simulink model "SD2231_Lab1_2024_final"  (R2023a)
settings: Solver=FixedStepAuto  StartTime=0.0  StopTime=inf  FixedStep=0.001  RelTol=1e-3  EnableMultiTasking=on
values from neighbouring files (symbols this model uses):
  K_brake = K_brake(3)    [initial_student.m]    (also in initial_student_final.m)
  K_em = K_em(3)    [initial_student.m]    (also in initial_student_final.m)
undefined symbols (not defined in the file or in its folder): DiscIntNeverNeededParam, Veh
libraries: CarMaker4SL x37, simulink x11, SignalEditorBlockLib x2, autolibmappedmotor x2
(part 2 of 4)

== system SD2231_Lab1_2024_final/CarMaker/Your ABS Controller/PID Controller ==
  <FL Braking Slip> : Inport
  <RL Braking Slip> : Inport  Port=2
  <Brake pedal> : Inport  Port=3
  Vehicle_Velocity : Inport  Port=4
  PID_Front_Breaking : Subsystem
  PID_Rear_Breaking : Subsystem
  Sum : Sum  Inputs=|-+
  Sum1 : Sum  Inputs=+-|
  Switch : Switch  Criteria=u2 > Threshold  Threshold=2.5  SaturateOnIntegerOverflow=off  InputSameDT=off
  Switch1 : Switch  Criteria=u2 > Threshold  Threshold=0.05  SaturateOnIntegerOverflow=off  InputSameDT=off
  Switch2 : Switch  Criteria=u2 > Threshold  Threshold=2.5  SaturateOnIntegerOverflow=off  InputSameDT=off
  Switch3 : Switch  Criteria=u2 > Threshold  Threshold=0.05  SaturateOnIntegerOverflow=off  InputSameDT=off
  Front_Braking : Outport
  Rear_Braking : Outport  Port=2
  wires:
  <FL Braking Slip>/1 -> PID_Front_Breaking/1(In1), Switch1/2
  PID_Front_Breaking/1(Out1) -> Sum/1
  <Brake pedal>/1 -> Switch3/3, Switch2/3, Switch1/3, Switch/3, Sum/2, Sum1/1
  <RL Braking Slip>/1 -> PID_Rear_Breaking/1(In1), Switch3/2
  Sum/1 -> Switch1/1
  Switch1/1 -> Switch/1
  Switch/1 -> Front_Braking/1
  Vehicle_Velocity/1 -> Switch/2, Switch2/2
  Switch3/1 -> Switch2/1
  Switch2/1 -> Rear_Braking/1
  Sum1/1 -> Switch3/1
  PID_Rear_Breaking/1(Out1) -> Sum1/2

== system SD2231_Lab1_2024_final/CarMaker/Your ABS Controller/PID Controller Advanced filter ==
  <FL Braking Slip> : Inport
  <RL Braking Slip> : Inport  Port=2
  <Brake pedal> : Inport  Port=3
  Vehicle_Velocity : Inport  Port=4
  PID_Front_Breaking : Subsystem
  PID_Rear_Breaking : Subsystem
  Sum : Sum  Inputs=|-+
  Sum1 : Sum  Inputs=+-|
  Switch : Switch  Criteria=u2 > Threshold  Threshold=2.5  SaturateOnIntegerOverflow=off  InputSameDT=off
  Switch1 : Switch  Criteria=u2 > Threshold  Threshold=0.05  SaturateOnIntegerOverflow=off  InputSameDT=off
  Switch2 : Switch  Criteria=u2 > Threshold  Threshold=2.5  SaturateOnIntegerOverflow=off  InputSameDT=off
  Switch3 : Switch  Criteria=u2 > Threshold  Threshold=0.05  SaturateOnIntegerOverflow=off  InputSameDT=off
  Front_Braking : Outport
  Rear_Braking : Outport  Port=2
  wires:
  <FL Braking Slip>/1 -> PID_Front_Breaking/1(In1), Switch1/2
  PID_Front_Breaking/1(Out1) -> Sum/1
  <Brake pedal>/1 -> Switch3/3, Switch2/3, Switch1/3, Switch/3, Sum/2, Sum1/1
  <RL Braking Slip>/1 -> PID_Rear_Breaking/1(In1), Switch3/2
  Sum/1 -> Switch1/1
  Switch1/1 -> Switch/1
  Switch/1 -> Front_Braking/1
  Vehicle_Velocity/1 -> Switch/2, Switch2/2
  Switch3/1 -> Switch2/1
  Switch2/1 -> Rear_Braking/1
  Sum1/1 -> Switch3/1
  PID_Rear_Breaking/1(Out1) -> Sum1/2

== system SD2231_Lab1_2024_final/CarMaker/Your ABS Controller/PID Controller windup ==
  <FL Braking Slip> : Inport
  <RL Braking Slip> : Inport  Port=2
  <Brake pedal> : Inport  Port=3
  Vehicle_Velocity : Inport  Port=4
  Minus : Sum  Inputs=+-
  Minus1 : Sum  Inputs=+-
  PID_Front_Breaking : Subsystem
  PID_Rear_Breaking : Subsystem
  Saturation : Saturate  UpperLimit=1  LowerLimit=0
  Saturation1 : Saturate  UpperLimit=1  LowerLimit=0
  Sum : Sum  Inputs=|-+
  Sum1 : Sum  Inputs=+-|
  Switch : Switch  Criteria=u2 > Threshold  Threshold=2.5  SaturateOnIntegerOverflow=off  InputSameDT=off
  Switch1 : Switch  Criteria=u2 > Threshold  Threshold=0.05  SaturateOnIntegerOverflow=off  InputSameDT=off
  Switch2 : Switch  Criteria=u2 > Threshold  Threshold=2.5  SaturateOnIntegerOverflow=off  InputSameDT=off
  Switch3 : Switch  Criteria=u2 > Threshold  Threshold=0.05  SaturateOnIntegerOverflow=off  InputSameDT=off
  Front_Braking : Outport
  Rear_Braking : Outport  Port=2
  wires:
  <FL Braking Slip>/1 -> PID_Front_Breaking/1(In1), Switch1/2
  PID_Front_Breaking/1(Out1) -> Sum/1
  <Brake pedal>/1 -> Switch3/3, Switch2/3, Switch1/3, Switch/3, Sum/2, Sum1/1
  <RL Braking Slip>/1 -> PID_Rear_Breaking/1(In1), Switch3/2
  Switch1/1 -> Switch/1
  Switch/1 -> Front_Braking/1
  Vehicle_Velocity/1 -> Switch/2, Switch2/2
  Switch3/1 -> Switch2/1
  Switch2/1 -> Rear_Braking/1
  Sum1/1 -> Saturation1/1, Minus1/2, Switch3/1
  PID_Rear_Breaking/1(Out1) -> Sum1/2
  Saturation/1 -> Minus/1
  Sum/1 -> Saturation/1, Minus/2, Switch1/1
  Minus/1 -> PID_Front_Breaking/2(In2)
  Saturation1/1 -> Minus1/1
  Minus1/1 -> PID_Rear_Breaking/2(In2)

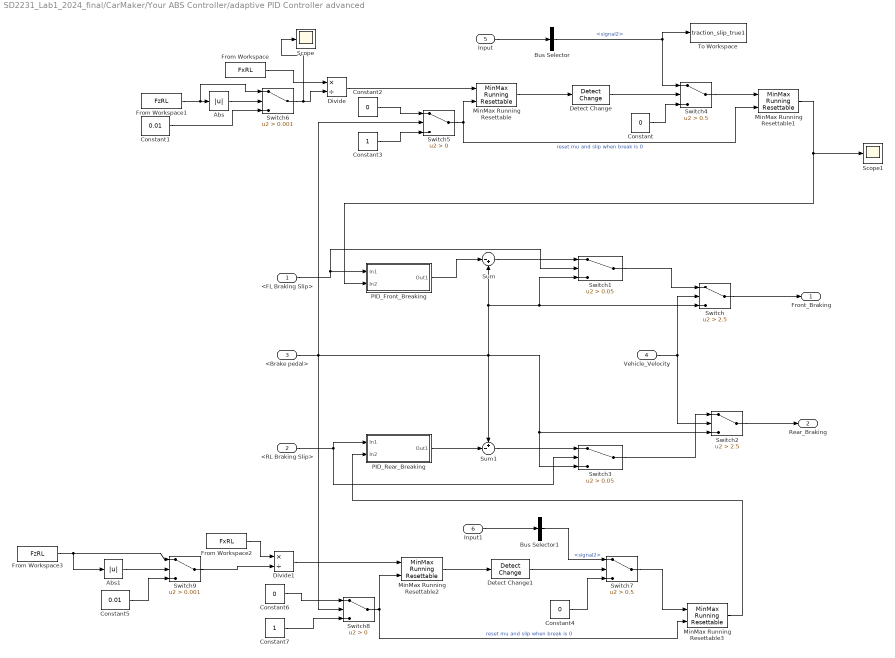
== system SD2231_Lab1_2024_final/CarMaker/Your ABS Controller/adaptive PID Controller advanced ==
  <FL Braking Slip> : Inport
  <RL Braking Slip> : Inport  Port=2
  <Brake pedal> : Inport  Port=3
  Vehicle_Velocity : Inport  Port=4
  Input : Inport  Port=5
  Input1 : Inport  Port=6
  Abs : Abs  SaturateOnIntegerOverflow=off
  Abs1 : Abs  SaturateOnIntegerOverflow=off
  Bus Selector : BusSelector  OutputSignals=signal2
  Bus Selector1 : BusSelector  OutputSignals=signal2
  Constant{,2,4,6} (4 alike) : Constant  Value=0
  Constant1 : Constant  Value=0.01
  Constant3 : Constant
  Constant5 : Constant  Value=0.01
  Constant7 : Constant
  Detect Change : simulink/Logic and Bit Operations/Detect Change  vinit=0  OutDataTypeStr=boolean
  Detect Change1 : simulink/Logic and Bit Operations/Detect Change  vinit=0  OutDataTypeStr=boolean
  Divide : Product  Inputs=*/
  Divide1 : Product  Inputs=*/
  From Workspace : FromWorkspace  VariableName=FxRL
  From Workspace1 : FromWorkspace  VariableName=FzRL
  From Workspace2 : FromWorkspace  VariableName=FxRL
  From Workspace3 : FromWorkspace  VariableName=FzRL
  MinMax Running Resettable : simulink/Math Operations/MinMax Running Resettable  Function=max  vinit=0.0
  MinMax Running Resettable1 : simulink/Math Operations/MinMax Running Resettable  Function=max  vinit=0.1
  MinMax Running Resettable2 : simulink/Math Operations/MinMax Running Resettable  Function=max  vinit=0.0
  MinMax Running Resettable3 : simulink/Math Operations/MinMax Running Resettable  Function=max  vinit=0.1
  PID_Front_Breaking : Subsystem
  PID_Rear_Breaking : Subsystem
  Scope : Scope
  Scope1 : Scope
  Sum : Sum  Inputs=|-+
  Sum1 : Sum  Inputs=+-|
  Switch : Switch  Criteria=u2 > Threshold  Threshold=2.5  SaturateOnIntegerOverflow=off  InputSameDT=off
  Switch1 : Switch  Criteria=u2 > Threshold  Threshold=0.05  SaturateOnIntegerOverflow=off  InputSameDT=off
  Switch2 : Switch  Criteria=u2 > Threshold  Threshold=2.5  SaturateOnIntegerOverflow=off  InputSameDT=off
  Switch3 : Switch  Criteria=u2 > Threshold  Threshold=0.05  SaturateOnIntegerOverflow=off  InputSameDT=off
  Switch4 : Switch  Criteria=u2 > Threshold  Threshold=0.5  SaturateOnIntegerOverflow=off  InputSameDT=off
  Switch5 : Switch  Criteria=u2 > Threshold  SaturateOnIntegerOverflow=off  InputSameDT=off
  Switch6 : Switch  Criteria=u2 > Threshold  Threshold=0.001  SaturateOnIntegerOverflow=off  InputSameDT=off
  Switch7 : Switch  Criteria=u2 > Threshold  Threshold=0.5  SaturateOnIntegerOverflow=off  InputSameDT=off
  Switch8 : Switch  Criteria=u2 > Threshold  SaturateOnIntegerOverflow=off  InputSameDT=off
  Switch9 : Switch  Criteria=u2 > Threshold  Threshold=0.001  SaturateOnIntegerOverflow=off  InputSameDT=off
  To Workspace : ToWorkspace  VariableName=traction_slip_true1  SaveFormat=Timeseries  SampleTime=-1
  Front_Braking : Outport
  Rear_Braking : Outport  Port=2
  wires:
  <FL Braking Slip>/1 -> PID_Front_Breaking/1(In1), Switch1/2
  PID_Front_Breaking/1(Out1) -> Sum/1
  <RL Braking Slip>/1 -> PID_Rear_Breaking/1(In1), Switch3/2
  Sum/1 -> Switch1/1
  Switch1/1 -> Switch/1
  Switch/1 -> Front_Braking/1
  Vehicle_Velocity/1 -> Switch/2, Switch2/2
  Switch3/1 -> Switch2/1
  Switch2/1 -> Rear_Braking/1
  Sum1/1 -> Switch3/1
  PID_Rear_Breaking/1(Out1) -> Sum1/2
  Abs/1 -> Switch6/2
  Switch6/1 -> Scope/1, Divide/2
  From Workspace1/1 -> Switch6/1, Abs/1
  Input/1 -> Bus Selector/1
  Constant/1 -> Switch4/3
  Bus Selector/1 -> To Workspace/1, Switch4/1  "<signal2>"
  From Workspace/1 -> Divide/1
  MinMax Running Resettable1/1 -> PID_Front_Breaking/2(In2), Scope1/1
  Constant1/1 -> Switch6/3
  MinMax Running Resettable/1 -> Detect Change/1
  Switch4/1 -> MinMax Running Resettable1/1
  Constant3/1 -> Switch5/3
  Switch5/1 -> MinMax Running Resettable/2, MinMax Running Resettable1/2  "reset mu and slip when break is 0"
  Constant2/1 -> Switch5/1
  Divide/1 -> MinMax Running Resettable/1
  Detect Change/1 -> Switch4/2
  Switch9/1 -> Divide1/2
  Abs1/1 -> Switch9/2
  Divide1/1 -> MinMax Running Resettable2/1
  Detect Change1/1 -> Switch7/2
  MinMax Running Resettable2/1 -> Detect Change1/1
  Constant7/1 -> Switch8/3
  Constant5/1 -> Switch9/3
  Switch7/1 -> MinMax Running Resettable3/1
  Constant6/1 -> Switch8/1
  Switch8/1 -> MinMax Running Resettable2/2, MinMax Running Resettable3/2  "reset mu and slip when break is 0"
  From Workspace2/1 -> Divide1/1
  Bus Selector1/1 -> Switch7/1  "<signal2>"
  Constant4/1 -> Switch7/3
  Input1/1 -> Bus Selector1/1
  <Brake pedal>/1 -> Switch5/2, Switch3/3, Switch2/3, Switch1/3, Switch/3, Sum/2, Sum1/1, Switch8/2
  From Workspace3/1 -> Abs1/1, Switch9/1
  MinMax Running Resettable3/1 -> PID_Rear_Breaking/2(In2)

== system SD2231_Lab1_2024_final/CarMaker/Your Traction Controller/P Controller ==
  <RL traction slip> : Inport
  <Throttle> : Inport  Port=2
  Vehicle_Velocity : Inport  Port=3
  P_Front_Breaking : Subsystem
  Sum : Sum  Inputs=|-+
  Switch : Switch  Criteria=u2 > Threshold  Threshold=2.5  SaturateOnIntegerOverflow=off  InputSameDT=off
  Switch1 : Switch  Criteria=u2 > Threshold  Threshold=0.3  SaturateOnIntegerOverflow=off  InputSameDT=off
  Throttle : Outport
  wires:
  <RL traction slip>/1 -> P_Front_Breaking/1(In1), Switch1/2
  P_Front_Breaking/1(Out1) -> Sum/1
  <Throttle>/1 -> Switch1/3, Switch/3, Sum/2
  Sum/1 -> Switch1/1
  Switch1/1 -> Switch/1
  Switch/1 -> Throttle/1
  Vehicle_Velocity/1 -> Switch/2

== system SD2231_Lab1_2024_final/CarMaker/Your Traction Controller/PD Controller ==
  <RL traction slip> : Inport
  <Throttle> : Inport  Port=2
  Vehicle_Velocity : Inport  Port=3
  P_Front_Breaking : Subsystem
  Sum : Sum  Inputs=|-+
  Switch : Switch  Criteria=u2 > Threshold  Threshold=2.5  SaturateOnIntegerOverflow=off  InputSameDT=off
  Switch1 : Switch  Criteria=u2 > Threshold  Threshold=0.3  SaturateOnIntegerOverflow=off  InputSameDT=off
  Throttle : Outport
  wires:
  <RL traction slip>/1 -> P_Front_Breaking/1(In1), Switch1/2
  P_Front_Breaking/1(Out1) -> Sum/1
  <Throttle>/1 -> Switch1/3, Switch/3, Sum/2
  Sum/1 -> Switch1/1
  Switch1/1 -> Switch/1
  Switch/1 -> Throttle/1
  Vehicle_Velocity/1 -> Switch/2

== system SD2231_Lab1_2024_final/CarMaker/Your Traction Controller/PI Controller ==
  <RL traction slip> : Inport
  <Throttle> : Inport  Port=2
  Vehicle_Velocity : Inport  Port=3
  P_Front_Breaking : Subsystem
  Sum : Sum  Inputs=|-+
  Switch : Switch  Criteria=u2 > Threshold  Threshold=2.5  SaturateOnIntegerOverflow=off  InputSameDT=off
  Switch1 : Switch  Criteria=u2 > Threshold  Threshold=0.2  SaturateOnIntegerOverflow=off  InputSameDT=off
  Throttle : Outport
  wires:
  <RL traction slip>/1 -> P_Front_Breaking/1(In1), Switch1/2
  P_Front_Breaking/1(Out1) -> Sum/1
  <Throttle>/1 -> Switch1/3, Switch/3, Sum/2
  Sum/1 -> Switch1/1
  Switch1/1 -> Switch/1
  Switch/1 -> Throttle/1
  Vehicle_Velocity/1 -> Switch/2

== system SD2231_Lab1_2024_final/CarMaker/Your Traction Controller/PID Controller ==
  <RL traction slip> : Inport
  <Throttle> : Inport  Port=2
  Vehicle_Velocity : Inport  Port=3
  P_Front_Breaking : Subsystem
  Sum : Sum  Inputs=|-+
  Switch : Switch  Criteria=u2 > Threshold  Threshold=2.5  SaturateOnIntegerOverflow=off  InputSameDT=off
  Switch1 : Switch  Criteria=u2 > Threshold  Threshold=0.2  SaturateOnIntegerOverflow=off  InputSameDT=off
  Throttle : Outport
  wires:
  <RL traction slip>/1 -> P_Front_Breaking/1(In1), Switch1/2
  P_Front_Breaking/1(Out1) -> Sum/1
  <Throttle>/1 -> Switch1/3, Switch/3, Sum/2
  Sum/1 -> Switch1/1
  Switch1/1 -> Switch/1
  Switch/1 -> Throttle/1
  Vehicle_Velocity/1 -> Switch/2

== system SD2231_Lab1_2024_final/CarMaker/Your Traction Controller/PID Controller Advanced anti-windup ==
  <RL traction slip> : Inport
  <Throttle> : Inport  Port=2
  Vehicle_Velocity : Inport  Port=3
  Minus : Sum  Inputs=+-
  P_Front_Breaking : Subsystem
  Saturation : Saturate  UpperLimit=1  LowerLimit=0
  Sum : Sum  Inputs=|-+
  Switch : Switch  Criteria=u2 > Threshold  Threshold=2.5  SaturateOnIntegerOverflow=off  InputSameDT=off
  Switch1 : Switch  Criteria=u2 > Threshold  Threshold=0.2  SaturateOnIntegerOverflow=off  InputSameDT=off
  Throttle : Outport
  wires:
  <RL traction slip>/1 -> P_Front_Breaking/1(In1), Switch1/2
  P_Front_Breaking/1(Out1) -> Sum/1
  <Throttle>/1 -> Switch1/3, Switch/3, Sum/2
  Sum/1 -> Minus/2, Switch1/1, Saturation/1
  Switch1/1 -> Switch/1
  Switch/1 -> Throttle/1
  Vehicle_Velocity/1 -> Switch/2
  Saturation/1 -> Minus/1
  Minus/1 -> P_Front_Breaking/2(In2)

== system SD2231_Lab1_2024_final/CarMaker/Your Traction Controller/PID Controller Advanced_filter ==
  <RL traction slip> : Inport
  <Throttle> : Inport  Port=2
  Vehicle_Velocity : Inport  Port=3
  P_Front_Breaking : Subsystem
  Sum : Sum  Inputs=|-+
  Switch : Switch  Criteria=u2 > Threshold  Threshold=2.5  SaturateOnIntegerOverflow=off  InputSameDT=off
  Switch1 : Switch  Criteria=u2 > Threshold  Threshold=0.2  SaturateOnIntegerOverflow=off  InputSameDT=off
  Throttle : Outport
  wires:
  <RL traction slip>/1 -> P_Front_Breaking/1(In1), Switch1/2
  P_Front_Breaking/1(Out1) -> Sum/1
  <Throttle>/1 -> Switch1/3, Switch/3, Sum/2
  Sum/1 -> Switch1/1
  Switch1/1 -> Switch/1
  Switch/1 -> Throttle/1
  Vehicle_Velocity/1 -> Switch/2

== system SD2231_Lab1_2024_final/CarMaker/Your Traction Controller/adaptive PID Controller Advanced ==
  <RL traction slip> : Inport
  <Throttle> : Inport  Port=2
  Vehicle_Velocity : Inport  Port=3
  Input : Inport  Port=4
  Abs : Abs  SaturateOnIntegerOverflow=off
  Bus Selector : BusSelector  OutputSignals=signal1
  Constant : Constant  Value=0
  Constant1 : Constant  Value=0.01
  Constant2 : Constant  Value=0
  Constant3 : Constant
  Detect Change : simulink/Logic and Bit Operations/Detect Change  vinit=0  OutDataTypeStr=boolean
  Divide : Product  Inputs=*/
  From Workspace : FromWorkspace  VariableName=FxRL
  From Workspace1 : FromWorkspace  VariableName=FzRL
  MinMax Running Resettable : simulink/Math Operations/MinMax Running Resettable  Function=max  vinit=0.0
  MinMax Running Resettable1 : simulink/Math Operations/MinMax Running Resettable  Function=max  vinit=0.1
  PID_Rear_Thrust : Subsystem
  Scope : Scope
  Scope1 : Scope
  Scope2 : Scope
  Sum : Sum  Inputs=|-+
  Switch : Switch  Criteria=u2 > Threshold  Threshold=2.5  SaturateOnIntegerOverflow=off  InputSameDT=off
  Switch1 : Switch  Criteria=u2 > Threshold  Threshold=0.2  SaturateOnIntegerOverflow=off  InputSameDT=off
  Switch2 : Switch  Criteria=u2 > Threshold  Threshold=0.5  SaturateOnIntegerOverflow=off  InputSameDT=off
  Switch3 : Switch  Criteria=u2 > Threshold  SaturateOnIntegerOverflow=off  InputSameDT=off
  Switch4 : Switch  Criteria=u2 > Threshold  Threshold=0.001  SaturateOnIntegerOverflow=off  InputSameDT=off
  To Workspace : ToWorkspace  VariableName=traction_slip_true  SaveFormat=Timeseries  SampleTime=-1
  To Workspace1 : ToWorkspace  VariableName=traction_slip_best  SaveFormat=Timeseries  SampleTime=-1
  Throttle : Outport
  wires:
  <RL traction slip>/1 -> Switch1/2, PID_Rear_Thrust/1(In1)
  PID_Rear_Thrust/1(Out1) -> Sum/1
  <Throttle>/1 -> Switch1/3, Switch/3, Sum/2, Switch3/2
  Sum/1 -> Switch1/1
  Switch1/1 -> Switch/1
  Switch/1 -> Throttle/1
  Vehicle_Velocity/1 -> Switch/2
  From Workspace/1 -> Divide/1
  Divide/1 -> MinMax Running Resettable/1
  MinMax Running Resettable/1 -> Detect Change/1
  Detect Change/1 -> Switch2/2
  Switch2/1 -> MinMax Running Resettable1/1
  Input/1 -> Bus Selector/1
  Bus Selector/1 -> To Workspace/1, Scope1/1, Switch2/1  "<signal1>"
  MinMax Running Resettable1/1 -> To Workspace1/1, PID_Rear_Thrust/2(adaptive reference), Scope2/1
  Constant2/1 -> Switch3/1
  Constant3/1 -> Switch3/3
  Switch3/1 -> MinMax Running Resettable/2, MinMax Running Resettable1/2  "reset mu and slip when throttle is 0"
  Constant/1 -> Switch2/3
  Switch4/1 -> Scope/1, Divide/2
  From Workspace1/1 -> Switch4/1, Abs/1
  Abs/1 -> Switch4/2
  Constant1/1 -> Switch4/3

== system SD2231_Lab1_2024_final/CarMaker/IPG Vehicle/Brake/CreateBus Vhcl.Wheel.PT ==
  In : Inport
  BusCreator1 : BusCreator  Inputs=20
  Demux1 : Demux  Outputs=20
      settings: DisplayOption=none
  Out : Outport  VectorParamsAs1DForOutWhenUnconnected=off
  wires:
  Demux1/20 -> BusCreator1/20  "Vhcl Trq_DriveSrc_trg d3"
  Demux1/19 -> BusCreator1/19  "Vhcl Trq_DriveSrc_trg d2"
  Demux1/18 -> BusCreator1/18  "Vhcl Trq_DriveSrc_trg d1"
  Demux1/17 -> BusCreator1/17  "Vhcl Trq_DriveSrc_trg d0"
  Demux1/16 -> BusCreator1/16  "Vhcl Wheel RR WhlBearing"
  Demux1/15 -> BusCreator1/15  "Vhcl Wheel RR Trq_T2W"
  Demux1/14 -> BusCreator1/14  "Vhcl Wheel RR Trq_BrakeReg_trg"
  Demux1/13 -> BusCreator1/13  "Vhcl Wheel RR Trq_Brake"
  Demux1/12 -> BusCreator1/12  "Vhcl Wheel RL WhlBearing"
  Demux1/11 -> BusCreator1/11  "Vhcl Wheel RL Trq_T2W"
  Demux1/10 -> BusCreator1/10  "Vhcl Wheel RL Trq_BrakeReg_trg"
  Demux1/9 -> BusCreator1/9  "Vhcl Wheel RL Trq_Brake"
  Demux1/8 -> BusCreator1/8  "Vhcl Wheel FR WhlBearing"
  Demux1/7 -> BusCreator1/7  "Vhcl Wheel FR Trq_T2W"
  Demux1/6 -> BusCreator1/6  "Vhcl Wheel FR Trq_BrakeReg_trg"
  Demux1/5 -> BusCreator1/5  "Vhcl Wheel FR Trq_Brake"
  Demux1/4 -> BusCreator1/4  "Vhcl Wheel FL WhlBearing"
  Demux1/3 -> BusCreator1/3  "Vhcl Wheel FL Trq_T2W"
  Demux1/2 -> BusCreator1/2  "Vhcl Wheel FL Trq_BrakeReg_trg"
  Demux1/1 -> BusCreator1/1  "Vhcl Wheel FL Trq_Brake"
  BusCreator1/1 -> Out/1
  In/1 -> Demux1/1

== system SD2231_Lab1_2024_final/CarMaker/IPG Vehicle/Brake/UserDefinedBrakingSystem ==
  note: Please note: Influence of DrivMan.Handbrake on the braking
      | torques (Brake IF Trq_XX signals) is ignored in this example.
  SD2231.Data : Inport
  Bus Creator2 : BusCreator  Inputs=16
  Bus Selector : BusSelector  OutputSignals=FLBrakeAdjust,FRBrakeAdjust,RLBrakeAdjust,RRBrakeAdjust
  Constant : Constant  Value=0
  NOTSET : Constant  Value=-99999
  Subsystem : Subsystem
  Subsystem1 : Subsystem
  Subsystem2 : Subsystem
  Subsystem3 : Subsystem
  Brake.IF.Out : Outport  VectorParamsAs1DForOutWhenUnconnected=off
  wires:
  SD2231.Data/1 -> Bus Selector/1
  Bus Creator2/1 -> Brake.IF.Out/1
  Constant/1 -> Bus Creator2/10, Bus Creator2/5, Bus Creator2/6, Bus Creator2/7, Bus Creator2/8, Bus Creator2/9, Bus Creator2/11, Bus Creator2/12
  NOTSET/1 -> Bus Creator2/13, Bus Creator2/14, Bus Creator2/15, Bus Creator2/16
  Subsystem/1(FL brake force) -> Bus Creator2/1
  Bus Selector/1 -> Subsystem/1(FLBrakeAdjust)  "<FLBrakeAdjust>"
  Subsystem1/1(FR brake force) -> Bus Creator2/2
  Subsystem2/1(RL brake force) -> Bus Creator2/3
  Subsystem3/1(RR brake force) -> Bus Creator2/4
  Bus Selector/2 -> Subsystem1/1(FRBrakeAdjust)  "<FRBrakeAdjust>"
  Bus Selector/3 -> Subsystem2/1(RLBrakeAdjust)  "<RLBrakeAdjust>"
  Bus Selector/4 -> Subsystem3/1(RRBrakeAdjust)  "<RRBrakeAdjust>"

== system SD2231_Lab1_2024_final/CarMaker/IPG Vehicle/CarAndTrailer/CarAndTrailerUpd ==
  Sync_In : Inport
  Vhcl.Steering : Inport  Port=2
  Vhcl.Motion : Inport  Port=3
  Vhcl.PoI : Inport  Port=4
  Vhcl.Wheel.FL : Inport  Port=5
  Vhcl.Wheel.FR : Inport  Port=6
  Vhcl.Wheel.RL : Inport  Port=7
  Vhcl.Wheel.RR : Inport  Port=8
  Car.Hitch.FrcTrq : Inport  Port=9
  Vhcl.Fr1A : Inport  Port=10
  CarAndTrailerUpd : S-Function  FunctionName=CM_Sfun  Parameters='CarAndTrUpd'  SFunctionDeploymentMode=off  EnableBusSupport=off
  CreateBus Brake.IF.In : Subsystem
  Sync_Out : Outport  VectorParamsAs1DForOutWhenUnconnected=off
  Brake.IF.In : Outport  Port=2  VectorParamsAs1DForOutWhenUnconnected=off
  wires:
  Vhcl.Fr1A/1 -> CarAndTrailerUpd/10  "user vehicle only"
  Vhcl.Steering/1 -> CarAndTrailerUpd/2
  Vhcl.Motion/1 -> CarAndTrailerUpd/3
  Vhcl.PoI/1 -> CarAndTrailerUpd/4
  Vhcl.Wheel.FL/1 -> CarAndTrailerUpd/5
  Vhcl.Wheel.FR/1 -> CarAndTrailerUpd/6
  Car.Hitch.FrcTrq/1 -> CarAndTrailerUpd/9
  Vhcl.Wheel.RR/1 -> CarAndTrailerUpd/8
  Vhcl.Wheel.RL/1 -> CarAndTrailerUpd/7
  CarAndTrailerUpd/2 -> CreateBus Brake.IF.In/1(In)
  CreateBus Brake.IF.In/1(Out) -> Brake.IF.In/1
  CarAndTrailerUpd/1 -> Sync_Out/1
  Sync_In/1 -> CarAndTrailerUpd/1

== system SD2231_Lab1_2024_final/CarMaker/IPG Vehicle/CarAndTrailer/Forces ==
  Sync_In : Inport
  TireFL_In : Inport  Port=2
  TireFR_In : Inport  Port=3
  TireRL_In : Inport  Port=4
  TireRR_In : Inport  Port=5
  lSpring : Inport  Port=6
  vDamp : Inport  Port=7
  lStabi : Inport  Port=8
  lBuf : Inport  Port=9
  External Suspension Forces : Subsystem
  Suspension Forces : Subsystem
  Tires : Subsystem
  Vehicle Forces : Subsystem
  Sync_Out : Outport  VectorParamsAs1DForOutWhenUnconnected=off
  Car.Virtual : Outport  Port=2  VectorParamsAs1DForOutWhenUnconnected=off
  Car.Aero : Outport  Port=3  VectorParamsAs1DForOutWhenUnconnected=off
  Car.Load : Outport  Port=4  VectorParamsAs1DForOutWhenUnconnected=off
  TireFL_Out : Outport  Port=5  VectorParamsAs1DForOutWhenUnconnected=off
  TireFR_Out : Outport  Port=6  VectorParamsAs1DForOutWhenUnconnected=off
  TireRL_Out : Outport  Port=7  VectorParamsAs1DForOutWhenUnconnected=off
  TireRR_Out : Outport  Port=8  VectorParamsAs1DForOutWhenUnconnected=off
  FSpring_ext : Outport  Port=9  VectorParamsAs1DForOutWhenUnconnected=off
  FDamp_ext : Outport  Port=10  VectorParamsAs1DForOutWhenUnconnected=off
  FStabi_ext : Outport  Port=11  VectorParamsAs1DForOutWhenUnconnected=off
  FBuf_ext : Outport  Port=12  VectorParamsAs1DForOutWhenUnconnected=off
  wires:
  lBuf/1 -> External Suspension Forces/5(lBuf), Suspension Forces/5(lBuf)
  lStabi/1 -> External Suspension Forces/4(lStabi), Suspension Forces/4(lStabi)
  vDamp/1 -> External Suspension Forces/3(vDamp), Suspension Forces/3(vDamp)
  Tires/4(TireRR_Out) -> TireRR_Out/1
  Tires/3(TireRL_Out) -> TireRL_Out/1
  Tires/2(TireFR_Out) -> TireFR_Out/1
  Tires/1(TireFL_Out) -> TireFL_Out/1
  TireRR_In/1 -> Tires/5(TireRR_In)
  TireRL_In/1 -> Tires/4(TireRL_In)
  TireFR_In/1 -> Tires/3(TireFR_In)
  TireFL_In/1 -> Tires/2(TireFL_In)
  External Suspension Forces/4(FBuf_ext) -> FBuf_ext/1
  Sync_In/1 -> External Suspension Forces/1(Sync_In), Tires/1(Sync_In), Vehicle Forces/1(Sync_In)
  Vehicle Forces/1(Sync_Out) -> Suspension Forces/1(Sync_In)
  Vehicle Forces/2(Car.Virtual) -> Car.Virtual/1
  Vehicle Forces/3(Car.Aero) -> Car.Aero/1
  Vehicle Forces/4(Car.Load) -> Car.Load/1
  lSpring/1 -> External Suspension Forces/2(lSpring), Suspension Forces/2(lSpring)
  External Suspension Forces/2(FDamp_ext) -> FDamp_ext/1
  External Suspension Forces/3(FStabi_ext) -> FStabi_ext/1
  External Suspension Forces/1(FSpring_ext) -> FSpring_ext/1
  Suspension Forces/1(Sync_Out) -> Sync_Out/1

== system SD2231_Lab1_2024_final/CarMaker/IPG Vehicle/CarAndTrailer/Kinematics ==
  Sync_In : Inport
  Steer.IF : Inport  Port=2
  Kinematics : S-Function  FunctionName=CM_Sfun  Parameters='Kinematics'  SFunctionDeploymentMode=off  EnableBusSupport=off
  Sync_Out : Outport  VectorParamsAs1DForOutWhenUnconnected=off
  TireFL_In : Outport  Port=2  VectorParamsAs1DForOutWhenUnconnected=off
  TireFR_In : Outport  Port=3  VectorParamsAs1DForOutWhenUnconnected=off
  TireRL_In : Outport  Port=4  VectorParamsAs1DForOutWhenUnconnected=off
  TireRR_In : Outport  Port=5  VectorParamsAs1DForOutWhenUnconnected=off
  lSpring : Outport  Port=6  VectorParamsAs1DForOutWhenUnconnected=off
  vDamp : Outport  Port=7  VectorParamsAs1DForOutWhenUnconnected=off
  lStabi : Outport  Port=8  VectorParamsAs1DForOutWhenUnconnected=off
  lBuf : Outport  Port=9  VectorParamsAs1DForOutWhenUnconnected=off
  wires:
  Kinematics/9 -> lBuf/1
  Kinematics/8 -> lStabi/1
  Kinematics/2 -> TireFL_In/1
  Kinematics/3 -> TireFR_In/1
  Kinematics/4 -> TireRL_In/1
  Kinematics/5 -> TireRR_In/1
  Kinematics/6 -> lSpring/1
  Kinematics/7 -> vDamp/1
  Sync_In/1 -> Kinematics/1
  Kinematics/1 -> Sync_Out/1
  Steer.IF/1 -> Kinematics/2

== system SD2231_Lab1_2024_final/CarMaker/IPG Vehicle/CarAndTrailer/Kinetics ==
  Sync_In : Inport
  Car.Virtual : Inport  Port=2
  Car.Aero : Inport  Port=3
  Car.Load : Inport  Port=4
  TireFL.Out : Inport  Port=5
  TireFR.Out : Inport  Port=6
  TireRL.Out : Inport  Port=7
  TireRR.Out : Inport  Port=8
  FSpring_ext : Inport  Port=9
  FDamp_ext : Inport  Port=10
  FStabi_ext : Inport  Port=11
  FBuf_ext : Inport  Port=12
  Bus Creator : BusCreator  Inputs=4
  Bus Creator1 : BusCreator  Inputs=12
  Bus Creator2 : BusCreator  Inputs=6
  Bus Creator3 : BusCreator  Inputs=6
  Bus Creator4 : BusCreator  Inputs=4
  Demux : Demux  Outputs=12
      settings: DisplayOption=none
  Demux1 : Demux  Outputs=6
      settings: DisplayOption=none
  Demux2 : Demux  Outputs=6
      settings: DisplayOption=none
  Demux3 : Demux
      settings: DisplayOption=none
  Demux4 : Demux
      settings: DisplayOption=none
  Kinetics : S-Function  FunctionName=CM_Sfun  Parameters='Kinetics'  SFunctionDeploymentMode=off  EnableBusSupport=off
  Sync_Out : Outport  VectorParamsAs1DForOutWhenUnconnected=off
  Trailer.Load : Outport  Port=2  VectorParamsAs1DForOutWhenUnconnected=off
  Car.Hitch : Outport  Port=3  VectorParamsAs1DForOutWhenUnconnected=off
  Car.Fr1 : Outport  Port=4  VectorParamsAs1DForOutWhenUnconnected=off
  Car.Trq_T2W : Outport  Port=5  VectorParamsAs1DForOutWhenUnconnected=off
  WheelCarrier.Misc : Outport  Port=6  VectorParamsAs1DForOutWhenUnconnected=off
  wires:
  FBuf_ext/1 -> Kinetics/12
  Sync_In/1 -> Kinetics/1
  Kinetics/1 -> Sync_Out/1
  Car.Aero/1 -> Kinetics/3
  Car.Virtual/1 -> Kinetics/2
  Bus Creator1/1 -> Trailer.Load/1
  Demux/1 -> Bus Creator1/1  "Trailer Load_0 mass"
  Demux/2 -> Bus Creator1/2  "Trailer Load_0 tx"
  Demux/3 -> Bus Creator1/3  "Trailer Load_0 ty"
  Demux/4 -> Bus Creator1/4  "Trailer Load_0 tz"
  Kinetics/2 -> Demux/1
  Demux/5 -> Bus Creator1/5  "Trailer Load_1 mass"
  Demux/6 -> Bus Creator1/6  "Trailer Load_1 tx"
  Demux/7 -> Bus Creator1/7  "Trailer Load_1 ty"
  Demux/8 -> Bus Creator1/8  "Trailer Load_1 tz"
  Demux/9 -> Bus Creator1/9  "Trailer Load_2 mass"
  Demux/10 -> Bus Creator1/10  "Trailer Load_2 tx"
  Demux/11 -> Bus Creator1/11  "Trailer Load_2 ty"
  Demux/12 -> Bus Creator1/12  "Trailer Load_2 tz"
  Demux1/1 -> Bus Creator2/1  "Car Hitch tx"
  Demux1/2 -> Bus Creator2/2  "Car Hitch ty"
  Demux1/3 -> Bus Creator2/3  "Car Hitch tz"
  Demux1/4 -> Bus Creator2/4  "Car Hitch vx"
  Demux1/5 -> Bus Creator2/5  "Car Hitch vy"
  Demux1/6 -> Bus Creator2/6  "Car Hitch vz"
  Kinetics/3 -> Demux1/1
  Bus Creator2/1 -> Car.Hitch/1
  Demux2/1 -> Bus Creator3/1  "Car Fr1 rx"
  Demux2/2 -> Bus Creator3/2  "Car Fr1 ry"
  Demux2/3 -> Bus Creator3/3  "Car Fr1 rz"
  Demux2/4 -> Bus Creator3/4  "Car Fr1 rvx"
  Demux2/5 -> Bus Creator3/5  "Car Fr1 rvy"
  Demux2/6 -> Bus Creator3/6  "Car Fr1 rvz"
  Bus Creator3/1 -> Car.Fr1/1
  Kinetics/4 -> Demux2/1
  Car.Load/1 -> Kinetics/4
  Demux3/1 -> Bus Creator4/1  "car Susp FL GenInert2"
  Demux3/2 -> Bus Creator4/2  "car Susp FR GenInert2"
  Demux3/3 -> Bus Creator4/3  "car Susp FL GenFrc2"
  Demux3/4 -> Bus Creator4/4  "car Susp FR GenFrc2"
  Bus Creator4/1 -> WheelCarrier.Misc/1
  Bus Creator/1 -> Car.Trq_T2W/1
  Demux4/4 -> Bus Creator/4  "Car Trq_T2WRR"
  Demux4/3 -> Bus Creator/3  "Car Trq_T2WRL"
  Demux4/2 -> Bus Creator/2  "Car Trq_T2WFR"
  Demux4/1 -> Bus Creator/1  "Car Trq_T2WFL"
  TireFL.Out/1 -> Kinetics/5
  TireFR.Out/1 -> Kinetics/6
  TireRL.Out/1 -> Kinetics/7
  TireRR.Out/1 -> Kinetics/8
  FSpring_ext/1 -> Kinetics/9
  FDamp_ext/1 -> Kinetics/10
  FStabi_ext/1 -> Kinetics/11
  Kinetics/6 -> Demux3/1
  Kinetics/5 -> Demux4/1

== system SD2231_Lab1_2024_final/CarMaker/IPG Vehicle/CarAndTrailer/Steering ==
  note: When replacing the entire steering system,
      | be sure to disable the IPG steering model by using the steering
      | model 'Model Manager off' in the vehicle GUI.
  Sync_In : Inport
  VhclCtrl.Steering : Inport  Port=2
  Bus Creator1 : BusCreator  Inputs=16
  Bus Creator2 : BusCreator  Inputs=5
  Demux : Demux  Outputs=21
      settings: DisplayOption=none
  Steering : S-Function  FunctionName=CM_Sfun  Parameters='Steering'  SFunctionDeploymentMode=off  EnableBusSupport=off
  Terminator : Terminator
  Sync_Out : Outport  VectorParamsAs1DForOutWhenUnconnected=off
  Steer.IF : Outport  Port=2  VectorParamsAs1DForOutWhenUnconnected=off
  wires:
  Demux/21 -> Bus Creator2/5  "Steering IF R Inert"
  Demux/20 -> Bus Creator2/4  "Steering IF R Frc"
  Demux/19 -> Bus Creator2/3  "Steering IF L Inert"
  Demux/18 -> Bus Creator2/2  "Steering IF L Frc"
  Demux/17 -> Bus Creator2/1  "Steering IF SteerByTrq"
  Demux/16 -> Bus Creator1/16  "Steering IF R iSteer2q"
  Demux/15 -> Bus Creator1/15  "Steering IF R qpp"
  Demux/14 -> Bus Creator1/14  "Steering IF R qp"
  Demux/13 -> Bus Creator1/13  "Steering IF R q"
  Demux/12 -> Bus Creator1/12  "Steering IF L iSteer2q"
  Demux/11 -> Bus Creator1/11  "Steering IF L qpp"
  Demux/10 -> Bus Creator1/10  "Steering IF L qp"
  Demux/9 -> Bus Creator1/9  "Steering IF L q"
  Demux/8 -> Bus Creator1/8  "Steering IF AssistTrqPin"
  Demux/7 -> Bus Creator1/7  "Steering IF AssistTrqCol"
  Demux/6 -> Bus Creator1/6  "Steering IF AssistFrc"
  Demux/5 -> Bus Creator1/5  "Steering IF TrqStatic"
  Demux/4 -> Bus Creator1/4  "Steering IF Trq"
  Demux/3 -> Bus Creator1/3  "Steering IF AngAcc"
  Demux/2 -> Bus Creator1/2  "Steering IF AngVel"
  Demux/1 -> Bus Creator1/1  "Steering IF Ang"
  Bus Creator1/1 -> Steer.IF/1
  Steering/2 -> Demux/1
  Bus Creator2/1 -> Terminator/1  "Steer IF (in)"
  VhclCtrl.Steering/1 -> Steering/2
  Steering/1 -> Sync_Out/1
  Sync_In/1 -> Steering/1

== system SD2231_Lab1_2024_final/CarMaker/IPG Vehicle/CarAndTrailer/Trailer ==
  Sync_In : Inport
  Trailer.Load : Inport  Port=2
  Car.Hitch : Inport  Port=3
  Car.Fr1 : Inport  Port=4
  Car.Trq_T2W : Inport  Port=5
  WheelCarrier.Misc : Inport  Port=6
  CreateBus Car.Hitch.FrcTrq : Subsystem
  CreateBus Vhcl.Motion : Subsystem
  CreateBus Vhcl.PoI : Subsystem
  CreateBus Vhcl.Steering : Subsystem
  CreateBus Vhcl.Wheel.FL : Subsystem
  CreateBus Vhcl.Wheel.FR : Subsystem
  CreateBus Vhcl.Wheel.RL : Subsystem
  CreateBus Vhcl.Wheel.RR : Subsystem
  Trailer : S-Function  FunctionName=CM_Sfun  Parameters='Trailer'  SFunctionDeploymentMode=off  EnableBusSupport=off
  Sync_Out : Outport  VectorParamsAs1DForOutWhenUnconnected=off
  Vhcl.Steering : Outport  Port=2  VectorParamsAs1DForOutWhenUnconnected=off
  Vhcl.Motion : Outport  Port=3  VectorParamsAs1DForOutWhenUnconnected=off
  Vhcl.PoI : Outport  Port=4  VectorParamsAs1DForOutWhenUnconnected=off
  Vhcl.Wheel.FL : Outport  Port=5  VectorParamsAs1DForOutWhenUnconnected=off
  Vhcl.Wheel.FR : Outport  Port=6  VectorParamsAs1DForOutWhenUnconnected=off
  Vhcl.Wheel.RL : Outport  Port=7  VectorParamsAs1DForOutWhenUnconnected=off
  Vhcl.Wheel.RR : Outport  Port=8  VectorParamsAs1DForOutWhenUnconnected=off
  Car.Hitch.FrcTrq : Outport  Port=9  VectorParamsAs1DForOutWhenUnconnected=off
  wires:
  Trailer/2 -> CreateBus Vhcl.Steering/1(In1)
  CreateBus Vhcl.Steering/1(Out1) -> Vhcl.Steering/1  "Vhcl.Steering"
  Trailer/3 -> CreateBus Vhcl.Motion/1(In1)
  Trailer/4 -> CreateBus Vhcl.PoI/1(In1)
  Trailer/5 -> CreateBus Vhcl.Wheel.FL/1(In1)
  Trailer/6 -> CreateBus Vhcl.Wheel.FR/1(In1)
  Trailer/7 -> CreateBus Vhcl.Wheel.RL/1(In1)
  Trailer/9 -> CreateBus Car.Hitch.FrcTrq/1(In1)
  Trailer/8 -> CreateBus Vhcl.Wheel.RR/1(In1)
  CreateBus Vhcl.Wheel.RR/1(Out1) -> Vhcl.Wheel.RR/1  "Vhcl.Wheel.RR"
  CreateBus Vhcl.Wheel.RL/1(Out1) -> Vhcl.Wheel.RL/1  "Vhcl.Wheel.RL"
  CreateBus Vhcl.Wheel.FR/1(Out1) -> Vhcl.Wheel.FR/1  "Vhcl.Wheel.FR"
  CreateBus Vhcl.Wheel.FL/1(Out1) -> Vhcl.Wheel.FL/1  "Vhcl.Wheel.FL"
  CreateBus Vhcl.PoI/1(Out1) -> Vhcl.PoI/1  "Vhcl.PoI"
  CreateBus Vhcl.Motion/1(Out1) -> Vhcl.Motion/1  "Vhcl.Motion"
  Car.Trq_T2W/1 -> Trailer/5
  WheelCarrier.Misc/1 -> Trailer/6
  CreateBus Car.Hitch.FrcTrq/1(Out1) -> Car.Hitch.FrcTrq/1  "Car.Hitch.FrcTrq"
  Car.Fr1/1 -> Trailer/4
  Car.Hitch/1 -> Trailer/3
  Trailer.Load/1 -> Trailer/2
  Trailer/1 -> Sync_Out/1
  Sync_In/1 -> Trailer/1

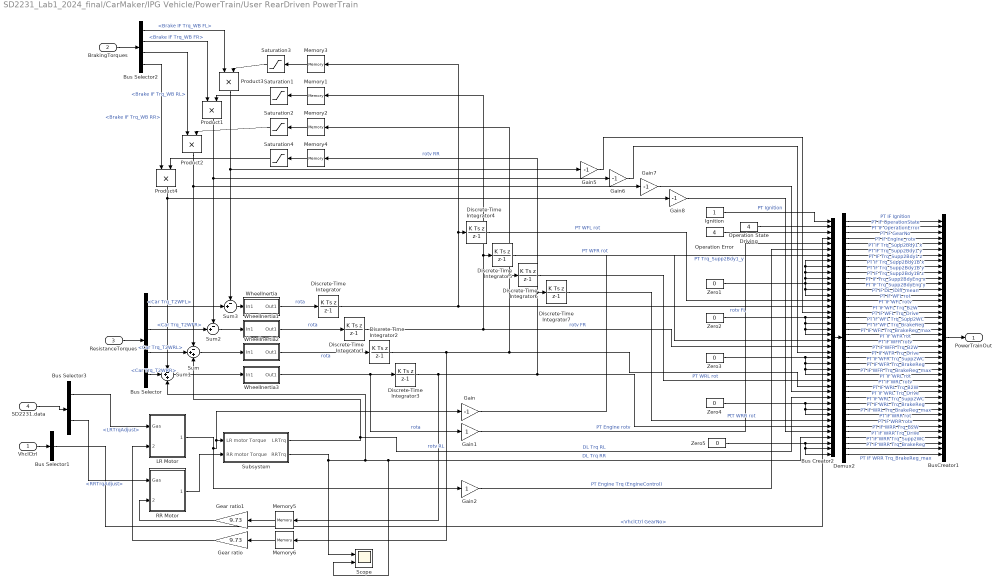
== system SD2231_Lab1_2024_final/CarMaker/IPG Vehicle/PowerTrain/User RearDriven PowerTrain ==
  VhclCtrl : Inport
  BrakingTorques : Inport  Port=2
  ResistanceTorques : Inport  Port=3
  SD2231.data : Inport  Port=4
  Bus Creator2 : BusCreator  Inputs=42
  Bus Selector : BusSelector  OutputSignals=Car Trq_T2WFL,Car Trq_T2WFR,Car Trq_T2WRL,Car Trq_T2WRR
  Bus Selector1 : BusSelector  OutputSignals=VhclCtrl GearNo
  Bus Selector2 : BusSelector  OutputSignals=Brake IF Trq_WB FL,Brake IF Trq_WB FR,Brake IF Trq_WB RL,Brake IF Trq_WB RR
  Bus Selector3 : BusSelector  OutputSignals=LRTrqAdjust,RRTrqAdjust
  BusCreator1 : BusCreator  Inputs=42
  Demux2 : Demux  Outputs=42
      settings: DisplayOption=none
  Discrete-Time Integrator{,1..7} (8 alike) : DiscreteIntegrator  IntegratorMethod=Integration: Backward Euler  SampleTime=0.001  ICPrevOutput=DiscIntNeverNeededParam  ICPrevScaledInput=DiscIntNeverNeededParam
  Gain{,5..8} (5 alike) : Gain  Gain=-1
      Gain settings: AttributesFormatString=%<Gain>
  Gain1 : Gain
      settings: AttributesFormatString=%<Gain>
  Gain2 : Gain
      settings: AttributesFormatString=%<Gain>
  Gear ratio : Gain  Gain=9.73
  Gear ratio1 : Gain  Gain=9.73
  Ignition : Constant
  LR Motor : Subsystem
  Memory{1..6} (6 alike) : Memory
  Operation Error : Constant  Value=4
  Operation State Driving : Constant  Value=4
  Product{1..4} (4 alike) : Product  RndMeth=Zero
  RR Motor : Subsystem
  Saturation{1..4} (4 alike) : Saturate  UpperLimit=1  LowerLimit=-1
  Scope : Scope  NumInputPorts=2
  Subsystem : Subsystem
  Sum : Sum  Inputs=-++
  Sum1 : Sum  Inputs=-++
  Sum2 : Sum  Inputs=-+|
  Sum3 : Sum  Inputs=-+|
  WheelInertia : Subsystem
  WheelInertia1 : Subsystem
  WheelInertia2 : Subsystem
  WheelInertia3 : Subsystem
  Zero{1..5} (5 alike) : Constant  Value=0
  PowerTrainOut : Outport  VectorParamsAs1DForOutWhenUnconnected=off
  wires:
  Saturation4/1 -> Product4/2
  Memory4/1 -> Saturation4/1
  Bus Selector2/4 -> Product4/1  "<Brake IF Trq_WB RR>"
  Product4/1 -> Sum1/1, Gain8/1
  Saturation2/1 -> Product2/2
  Memory2/1 -> Saturation2/1
  Bus Selector2/3 -> Product2/1  "<Brake IF Trq_WB RL>"
  Product2/1 -> Sum/1, Gain7/1
  Saturation1/1 -> Product1/2
  Memory1/1 -> Saturation1/1
  Bus Selector2/2 -> Product1/1  "<Brake IF Trq_WB FR>"
  Product1/1 -> Sum2/1, Gain6/1
  Memory3/1 -> Saturation3/1
  Saturation3/1 -> Product3/2
  Bus Selector2/1 -> Product3/1  "<Brake IF Trq_WB FL>"
  Product3/1 -> Sum3/1, Gain5/1
  BrakingTorques/1 -> Bus Selector2/1
  Sum3/1 -> WheelInertia/1(In1)
  Bus Selector/1 -> Sum3/2  "<Car Trq_T2WFL>"
  Sum2/1 -> WheelInertia1/1(In1)
  Bus Selector/4 -> Sum1/2  "<Car Trq_T2WRR>"
  Bus Selector/3 -> Sum/2  "<Car Trq_T2WRL>"
  Bus Selector1/1 -> Bus Creator2/4  "<VhclCtrl GearNo>"
  VhclCtrl/1 -> Bus Selector1/1
  LR Motor/1(Motor Trq) -> Gain2/1, Gain/1, Subsystem/1(LR motor Torque)
  Discrete-Time Integrator3/1 -> Memory5/1, Memory4/1, Discrete-Time Integrator7/1, Bus Creator2/37  "rotv RR"
  Discrete-Time Integrator/1 -> Memory3/1, Discrete-Time Integrator4/1, Bus Creator2/16  "rotv FL"
  Discrete-Time Integrator1/1 -> Memory1/1, Discrete-Time Integrator5/1, Bus Creator2/23  "rotv FR"
  Discrete-Time Integrator2/1 -> Memory6/1, Memory2/1, Discrete-Time Integrator6/1, Bus Creator2/30  "rotv RL"
  Sum1/1 -> WheelInertia3/1(In1)
  WheelInertia3/1(Out1) -> Gain1/1, Discrete-Time Integrator3/1  "rota"
  Sum/1 -> WheelInertia2/1(In1)
  WheelInertia2/1(Out1) -> Discrete-Time Integrator2/1  "rota"
  Bus Selector/2 -> Sum2/2  "<Car Trq_T2WFR>"
  WheelInertia1/1(Out1) -> Discrete-Time Integrator1/1  "rota"
  ResistanceTorques/1 -> Bus Selector/1
  WheelInertia/1(Out1) -> Discrete-Time Integrator/1  "rota"
  Gain/1 -> Bus Creator2/7  "PT Trq_Supp2Bdy1_y"
  Gain1/1 -> Bus Creator2/5  "PT Engine rotv"
  Gain2/1 -> Bus Creator2/6  "PT Engine Trq (EngineControl)"
  Discrete-Time Integrator7/1 -> Bus Creator2/36  "PtT WRR rot"
  Discrete-Time Integrator6/1 -> Bus Creator2/29  "PT WRL rot"
  Discrete-Time Integrator5/1 -> Bus Creator2/22  "PT WFR rot"
  Discrete-Time Integrator4/1 -> Bus Creator2/15  "PT WFL rot"
  Ignition/1 -> Bus Creator2/1  "PT Ignition"
  Bus Creator2/1 -> Demux2/1
  Operation State Driving/1 -> Bus Creator2/2
  Operation Error/1 -> Bus Creator2/3
  Zero1/1 -> Bus Creator2/12, Bus Creator2/14, Bus Creator2/13, Bus Creator2/11, Bus Creator2/10, Bus Creator2/9, Bus Creator2/8
  Zero2/1 -> Bus Creator2/19, Bus Creator2/20, Bus Creator2/21, Bus Creator2/18
  Zero3/1 -> Bus Creator2/26, Bus Creator2/27, Bus Creator2/28, Bus Creator2/25
  Zero4/1 -> Bus Creator2/33, Bus Creator2/34, Bus Creator2/35
  Zero5/1 -> Bus Creator2/40, Bus Creator2/41, Bus Creator2/42
  Subsystem/1("LRTrq ") -> Bus Creator2/32, Sum/3  "DL Trq RL"
  Gain6/1 -> Bus Creator2/24
  Gain5/1 -> Bus Creator2/17
  Gain7/1 -> Bus Creator2/31
  Gain8/1 -> Bus Creator2/38
  Demux2/42 -> BusCreator1/42  "PT IF WRR Trq_BrakeReg_max"
  Demux2/41 -> BusCreator1/41  "PT IF WRR Trq_BrakeReg"
  Demux2/40 -> BusCreator1/40  "PT IF WRR Trq_Supp2WC"
  Demux2/39 -> BusCreator1/39  "PT IF WRR Trq_Drive"
  Demux2/38 -> BusCreator1/38  "PT IF WRR Trq_B2W"
  Demux2/37 -> BusCreator1/37  "PT IF WRR rotv"
  Demux2/36 -> BusCreator1/36  "PT IF WRR rot"
  Demux2/35 -> BusCreator1/35  "PT IF WRL Trq_BrakeReg_max"
  Demux2/34 -> BusCreator1/34  "PT IF WRL Trq_BrakeReg"
  Demux2/33 -> BusCreator1/33  "PT IF WRL Trq_Supp2WC"
  Demux2/32 -> BusCreator1/32  "PT IF WRL Trq_Drive"
  Demux2/31 -> BusCreator1/31  "PT IF WRL Trq_B2W"
  Demux2/30 -> BusCreator1/30  "PT IF WRL rotv"
  Demux2/29 -> BusCreator1/29  "PT IF WRL rot"
  Demux2/28 -> BusCreator1/28  "PT IF WFR Trq_BrakeReg_max"
  Demux2/27 -> BusCreator1/27  "PT IF WFR Trq_BrakeReg"
  Demux2/26 -> BusCreator1/26  "PT IF WFR Trq_Supp2WC"
  Demux2/25 -> BusCreator1/25  "PT IF WFR Trq_Drive"
  Demux2/24 -> BusCreator1/24  "PT IF WFR Trq_B2W"
  Demux2/23 -> BusCreator1/23  "PT IF WFR rotv"
  Demux2/22 -> BusCreator1/22  "PT IF WFR rot"
  Demux2/21 -> BusCreator1/21  "PT IF WFL Trq_BrakeReg_max"
  Demux2/20 -> BusCreator1/20  "PT IF WFL Trq_BrakeReg"
  Demux2/19 -> BusCreator1/19  "PT IF WFL Trq_Supp2WC"
  Demux2/18 -> BusCreator1/18  "PT IF WFL Trq_Drive"
  Demux2/17 -> BusCreator1/17  "PT IF WFL Trq_B2W"
  Demux2/16 -> BusCreator1/16  "PT IF WFL rotv"
  Demux2/15 -> BusCreator1/15  "PT IF WFL rot"
  Demux2/14 -> BusCreator1/14  "PT IF DL_iDiff_mean"
  Demux2/13 -> BusCreator1/13  "PT IF Trq_Supp2BdyEng y"
  Demux2/12 -> BusCreator1/12  "PT IF Trq_Supp2BdyEng x"
  Demux2/11 -> BusCreator1/11  "PT IF Trq_Supp2Bdy1B z"
  Demux2/10 -> BusCreator1/10  "PT IF Trq_Supp2Bdy1B y"
  Demux2/9 -> BusCreator1/9  "PT IF Trq_Supp2Bdy1B x"
  Demux2/8 -> BusCreator1/8  "PT IF Trq_Supp2Bdy1 z"
  Demux2/7 -> BusCreator1/7  "PT IF Trq_Supp2Bdy1 y"
  Demux2/6 -> BusCreator1/6  "PT IF Trq_Supp2Bdy1 x"
  Demux2/5 -> BusCreator1/5  "PT IF Engine_rotv"
  Demux2/4 -> BusCreator1/4  "PT IF GearNo"
  Demux2/3 -> BusCreator1/3  "PT IF OperationError"
  Demux2/2 -> BusCreator1/2  "PT IF OperationState"
  Demux2/1 -> BusCreator1/1  "PT IF Ignition"
  BusCreator1/1 -> PowerTrainOut/1
  Memory5/1 -> Gear ratio1/1
  Subsystem/2(RRTrq) -> Scope/1, Scope/2, Bus Creator2/39, Sum1/3  "DL Trq RR"
  SD2231.data/1 -> Bus Selector3/1
  Bus Selector3/1 -> LR Motor/1(Gas)  "<LRTrqAdjust>"
  RR Motor/1(Motor Trq) -> Subsystem/2(RR motor Torque)
  Bus Selector3/2 -> RR Motor/1(Gas)  "<RRTrqAdjust>"
  Memory6/1 -> Gear ratio/1
  Gear ratio/1 -> LR Motor/2("Motor speed ")
  Gear ratio1/1 -> RR Motor/2("Motor speed ")

== system SD2231_Lab1_2024_final/CarMaker/Your ABS Controller/P Controller/P_Front_Breaking ==
  In1 : Inport
  Constant : Constant  Value=0.05
  Derivative : Derivative
  Derivative Gain : Gain  Gain=0
  Integral Gain : Gain  Gain=0
  Integrator : Integrator
  Proportional Gain : Gain  Gain=-10
  Sum : Sum  Inputs=+++
  Sum1 : Sum  Inputs=|+-
  Out1 : Outport
  wires:
  Derivative Gain/1 -> Derivative/1
  Integral Gain/1 -> Integrator/1
  Integrator/1 -> Sum/2
  Sum/1 -> Out1/1
  Proportional Gain/1 -> Sum/1
  Derivative/1 -> Sum/3
  In1/1 -> Sum1/2
  Sum1/1 -> Integral Gain/1, Derivative Gain/1, Proportional Gain/1
  Constant/1 -> Sum1/1

== system SD2231_Lab1_2024_final/CarMaker/Your ABS Controller/P Controller/P_Rear_Breaking ==
  In1 : Inport
  Constant : Constant  Value=0.05
  Derivative : Derivative
  Derivative Gain : Gain  Gain=0
  Integral Gain : Gain  Gain=0
  Integrator : Integrator
  Proportional Gain : Gain  Gain=-10
  Sum : Sum  Inputs=+++
  Sum1 : Sum  Inputs=|+-
  Out1 : Outport
  wires:
  Derivative Gain/1 -> Derivative/1
  Integral Gain/1 -> Integrator/1
  Integrator/1 -> Sum/2
  Sum/1 -> Out1/1
  Proportional Gain/1 -> Sum/1
  Derivative/1 -> Sum/3
  In1/1 -> Sum1/2
  Sum1/1 -> Integral Gain/1, Derivative Gain/1, Proportional Gain/1
  Constant/1 -> Sum1/1

== system SD2231_Lab1_2024_final/CarMaker/Your ABS Controller/PD Controller/PD_Front_Breaking ==
  In1 : Inport
  Constant : Constant  Value=0.05
  Derivative : Derivative
  Derivative Gain : Gain  Gain=-0.001
  Integral Gain : Gain  Gain=0
  Integrator : Integrator  ExternalReset=falling
  Proportional Gain : Gain  Gain=-5
  Sum : Sum  Inputs=+++
  Sum1 : Sum  Inputs=|+-
  Out1 : Outport
  wires:
  Derivative Gain/1 -> Derivative/1
  Integral Gain/1 -> Integrator/1
  Integrator/1 -> Sum/2
  Sum/1 -> Out1/1
  Proportional Gain/1 -> Sum/1
  Derivative/1 -> Sum/3
  In1/1 -> Sum1/2
  Sum1/1 -> Derivative Gain/1, Integrator/2, Integral Gain/1, Proportional Gain/1
  Constant/1 -> Sum1/1

== system SD2231_Lab1_2024_final/CarMaker/Your ABS Controller/PD Controller/PD_Rear_Breaking ==
  In1 : Inport
  Constant : Constant  Value=0.05
  Derivative : Derivative
  Derivative Gain : Gain  Gain=-0.001
  Integral Gain : Gain  Gain=0
  Integrator : Integrator  ExternalReset=falling
  Proportional Gain : Gain  Gain=-5
  Sum : Sum  Inputs=+++
  Sum1 : Sum  Inputs=|+-
  Out1 : Outport
  wires:
  Derivative Gain/1 -> Derivative/1
  Integral Gain/1 -> Integrator/1
  Integrator/1 -> Sum/2
  Sum/1 -> Out1/1
  Proportional Gain/1 -> Sum/1
  Derivative/1 -> Sum/3
  In1/1 -> Sum1/2
  Sum1/1 -> Derivative Gain/1, Integrator/2, Integral Gain/1, Proportional Gain/1
  Constant/1 -> Sum1/1

== system SD2231_Lab1_2024_final/CarMaker/Your ABS Controller/PI Controller/PI_Front_Breaking ==
  In1 : Inport
  Constant : Constant  Value=0.05
  Derivative : Derivative
  Derivative Gain : Gain  Gain=0
  Integral Gain : Gain  Gain=-10
  Integrator : Integrator  ExternalReset=falling
  Proportional Gain : Gain  Gain=-8
  Sum : Sum  Inputs=+++
  Sum1 : Sum  Inputs=|+-
  Out1 : Outport
  wires:
  Derivative Gain/1 -> Derivative/1
  Integral Gain/1 -> Integrator/1
  Integrator/1 -> Sum/2
  Sum/1 -> Out1/1
  Proportional Gain/1 -> Sum/1
  Derivative/1 -> Sum/3
  In1/1 -> Sum1/2
  Sum1/1 -> Derivative Gain/1, Integrator/2, Integral Gain/1, Proportional Gain/1
  Constant/1 -> Sum1/1

== system SD2231_Lab1_2024_final/CarMaker/Your ABS Controller/PI Controller/PI_Rear_Breaking ==
  In1 : Inport
  Constant : Constant  Value=0.05
  Derivative : Derivative
  Derivative Gain : Gain  Gain=0
  Integral Gain : Gain  Gain=-10
  Integrator : Integrator  ExternalReset=falling
  Proportional Gain : Gain  Gain=-10
  Sum : Sum  Inputs=+++
  Sum1 : Sum  Inputs=|+-
  Out1 : Outport
  wires:
  Derivative Gain/1 -> Derivative/1
  Integral Gain/1 -> Integrator/1
  Integrator/1 -> Sum/2
  Sum/1 -> Out1/1
  Proportional Gain/1 -> Sum/1
  Derivative/1 -> Sum/3
  In1/1 -> Sum1/2
  Sum1/1 -> Derivative Gain/1, Integrator/2, Integral Gain/1, Proportional Gain/1
  Constant/1 -> Sum1/1

== system SD2231_Lab1_2024_final/CarMaker/Your ABS Controller/PID Controller/PID_Front_Breaking ==
  In1 : Inport
  Constant : Constant  Value=0.05
  Derivative : Derivative
  Derivative Gain : Gain  Gain=-0.001
  Integral Gain : Gain  Gain=-10
  Integrator : Integrator  ExternalReset=falling
  Proportional Gain : Gain  Gain=-6
  Sum : Sum  Inputs=+++
  Sum1 : Sum  Inputs=|+-
  Out1 : Outport
  wires:
  Derivative Gain/1 -> Derivative/1
  Integral Gain/1 -> Integrator/1
  Integrator/1 -> Sum/2
  Sum/1 -> Out1/1
  Proportional Gain/1 -> Sum/1
  Derivative/1 -> Sum/3
  In1/1 -> Sum1/2
  Sum1/1 -> Integrator/2, Derivative Gain/1, Integral Gain/1, Proportional Gain/1
  Constant/1 -> Sum1/1

== system SD2231_Lab1_2024_final/CarMaker/Your ABS Controller/PID Controller/PID_Rear_Breaking ==
  In1 : Inport
  Constant : Constant  Value=0.05
  Derivative : Derivative
  Derivative Gain : Gain  Gain=-0.001
  Integral Gain : Gain  Gain=-10
  Integrator : Integrator  ExternalReset=falling
  Proportional Gain : Gain  Gain=-6
  Sum : Sum  Inputs=+++
  Sum1 : Sum  Inputs=|+-
  Out1 : Outport
  wires:
  Derivative Gain/1 -> Derivative/1
  Integral Gain/1 -> Integrator/1
  Integrator/1 -> Sum/2
  Sum/1 -> Out1/1
  Proportional Gain/1 -> Sum/1
  Derivative/1 -> Sum/3
  In1/1 -> Sum1/2
  Sum1/1 -> Derivative Gain/1, Integrator/2, Integral Gain/1, Proportional Gain/1
  Constant/1 -> Sum1/1

== system SD2231_Lab1_2024_final/CarMaker/Your ABS Controller/PID Controller Advanced filter/PID_Front_Breaking ==
  In1 : Inport
  Constant : Constant  Value=0.05
  Derivative Gain : Gain  Gain=-0.001
  Gain : Gain  Gain=2
  Integral Gain : Gain  Gain=-10
  Integrator : Integrator  ExternalReset=falling
  Integrator1 : Integrator
  Proportional Gain : Gain  Gain=-6
  Sum : Sum  Inputs=+++
  Sum1 : Sum  Inputs=|+-
  Sum2 : Sum  Inputs=|+-
  Out1 : Outport
  wires:
  Integral Gain/1 -> Integrator/1
  Integrator/1 -> Sum/2
  Sum/1 -> Out1/1
  Proportional Gain/1 -> Sum/1
  In1/1 -> Sum1/2
  Sum1/1 -> Integrator/2, Derivative Gain/1, Integral Gain/1, Proportional Gain/1
  Constant/1 -> Sum1/1
  Derivative Gain/1 -> Sum2/1
  Sum2/1 -> Gain/1
  Integrator1/1 -> Sum2/2
  Gain/1 -> Sum/3, Integrator1/1

== system SD2231_Lab1_2024_final/CarMaker/Your ABS Controller/PID Controller Advanced filter/PID_Rear_Breaking ==
  In1 : Inport
  Constant : Constant  Value=0.05
  Derivative Gain : Gain  Gain=-0.001
  Gain : Gain  Gain=2
  Integral Gain : Gain  Gain=-10
  Integrator : Integrator  ExternalReset=falling
  Integrator1 : Integrator
  Proportional Gain : Gain  Gain=-6
  Sum : Sum  Inputs=+++
  Sum1 : Sum  Inputs=|+-
  Sum2 : Sum  Inputs=|+-
  Out1 : Outport
  wires:
  Integral Gain/1 -> Integrator/1
  Integrator/1 -> Sum/2
  Sum/1 -> Out1/1
  Proportional Gain/1 -> Sum/1
  In1/1 -> Sum1/2
  Sum1/1 -> Derivative Gain/1, Integrator/2, Integral Gain/1, Proportional Gain/1
  Constant/1 -> Sum1/1
  Sum2/1 -> Gain/1
  Gain/1 -> Sum/3, Integrator1/1
  Integrator1/1 -> Sum2/2
  Derivative Gain/1 -> Sum2/1

== system SD2231_Lab1_2024_final/CarMaker/Your ABS Controller/PID Controller windup/PID_Front_Breaking ==
  In1 : Inport
  In2 : Inport  Port=2
  Constant : Constant  Value=0.05
  Derivative : Derivative
  Derivative Gain : Gain  Gain=-0.001
  Integral Gain : Gain  Gain=-10
  Integrator : Integrator  ExternalReset=falling
  Proportional Gain : Gain  Gain=-6
  Sum : Sum  Inputs=+++
  Sum1 : Sum  Inputs=|+-
  Sum2 : Sum  Inputs=|++
  Out1 : Outport
  wires:
  Derivative Gain/1 -> Derivative/1
  Integrator/1 -> Sum/2
  Sum/1 -> Out1/1
  Proportional Gain/1 -> Sum/1
  Derivative/1 -> Sum/3
  In1/1 -> Sum1/2
  Sum1/1 -> Integrator/2, Derivative Gain/1, Integral Gain/1, Proportional Gain/1
  Constant/1 -> Sum1/1
  Sum2/1 -> Integrator/1
  Integral Gain/1 -> Sum2/1
  In2/1 -> Sum2/2

== system SD2231_Lab1_2024_final/CarMaker/Your ABS Controller/PID Controller windup/PID_Rear_Breaking ==
  In1 : Inport
  In2 : Inport  Port=2
  Constant : Constant  Value=0.05
  Derivative : Derivative
  Derivative Gain : Gain  Gain=-0.001
  Integral Gain : Gain  Gain=-10
  Integrator : Integrator  ExternalReset=falling
  Proportional Gain : Gain  Gain=-6
  Sum : Sum  Inputs=+++
  Sum1 : Sum  Inputs=|+-
  Sum2 : Sum  Inputs=|++
  Out1 : Outport
  wires:
  Derivative Gain/1 -> Derivative/1
  Integrator/1 -> Sum/2
  Sum/1 -> Out1/1
  Proportional Gain/1 -> Sum/1
  Derivative/1 -> Sum/3
  In1/1 -> Sum1/2
  Sum1/1 -> Derivative Gain/1, Integrator/2, Integral Gain/1, Proportional Gain/1
  Constant/1 -> Sum1/1
  In2/1 -> Sum2/2
  Integral Gain/1 -> Sum2/1
  Sum2/1 -> Integrator/1

== system SD2231_Lab1_2024_final/CarMaker/Your ABS Controller/adaptive PID Controller advanced/PID_Front_Breaking ==
  In1 : Inport
  In2 : Inport  Port=2
  Constant : Constant  Commented=on  Value=0.05
  Derivative : Derivative
  Derivative Gain : Gain  Gain=-0.001
  Integral Gain : Gain  Gain=-10
  Integrator : Integrator  ExternalReset=falling
  Proportional Gain : Gain  Gain=-6
  Sum : Sum  Inputs=+++
  Sum1 : Sum  Inputs=|+-
  Out1 : Outport
  wires:
  Derivative Gain/1 -> Derivative/1
  Integral Gain/1 -> Integrator/1
  Integrator/1 -> Sum/2
  Sum/1 -> Out1/1
  Proportional Gain/1 -> Sum/1
  Derivative/1 -> Sum/3
  In1/1 -> Sum1/2
  Sum1/1 -> Integrator/2, Derivative Gain/1, Integral Gain/1, Proportional Gain/1
  In2/1 -> Sum1/1
